simulink model "tanque_opcional"  (R2020b)
settings: Solver=VariableStepAuto  StartTime=0.0  StopTime=10000000  FixedStep=0.1  RelTol=1e-3
settings Model: Creator=Darkhorrow  LastModifiedBy=Darkhorrow

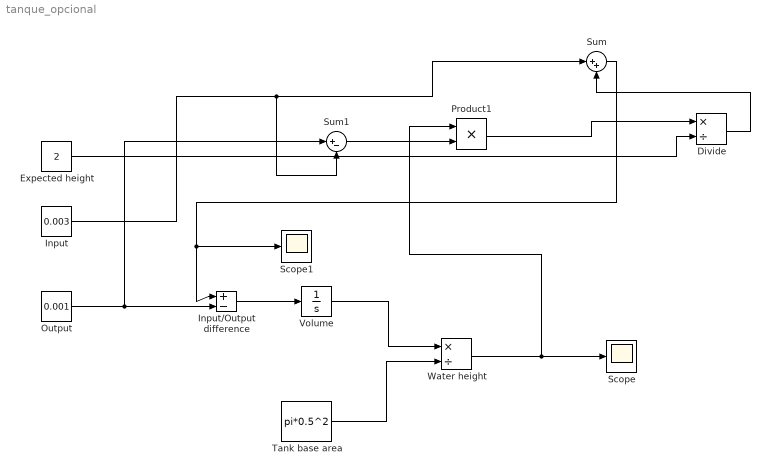
== system tanque_opcional ==
  Divide : Product  Inputs=*/
  Expected height : Constant  Value=2
  Input : Constant  Value=0.003
  Input/Output difference : Sum  Inputs=|+-
  Output : Constant  Value=0.001
  Product1 : Product
  Scope : Scope
  Scope1 : Scope
  Sum : Sum  Inputs=|++
  Sum1 : Sum  Inputs=|+-
  Tank base area : Constant  Value=pi*0.5^2
  Volume : Integrator
  Water height : Product  Inputs=*/
  wires:
  Volume/1 -> Water height/1
  Output/1 -> Sum1/1, Input/Output difference/2
  Input/1 -> Sum1/2, Sum/1
  Input/Output difference/1 -> Volume/1
  Tank base area/1 -> Water height/2
  Water height/1 -> Product1/1, Scope/1
  Product1/1 -> Divide/1
  Expected height/1 -> Divide/2
  Divide/1 -> Sum/2
  Sum/1 -> Input/Output difference/1, Scope1/1
  Sum1/1 -> Product1/2
